simulink model "DC_Charging_Sequence_Block_testing"  (R2024b)
settings: Solver=FixedStepDiscrete  StartTime=0.0  StopTime=10.0  FixedStep=0.01  RelTol=1e-3
undefined symbols (not defined in the file or in its folder): CCM, raptor_get_safe_string, raptor_xcp_function
libraries: Raptor_lib x37
(part 2 of 2)

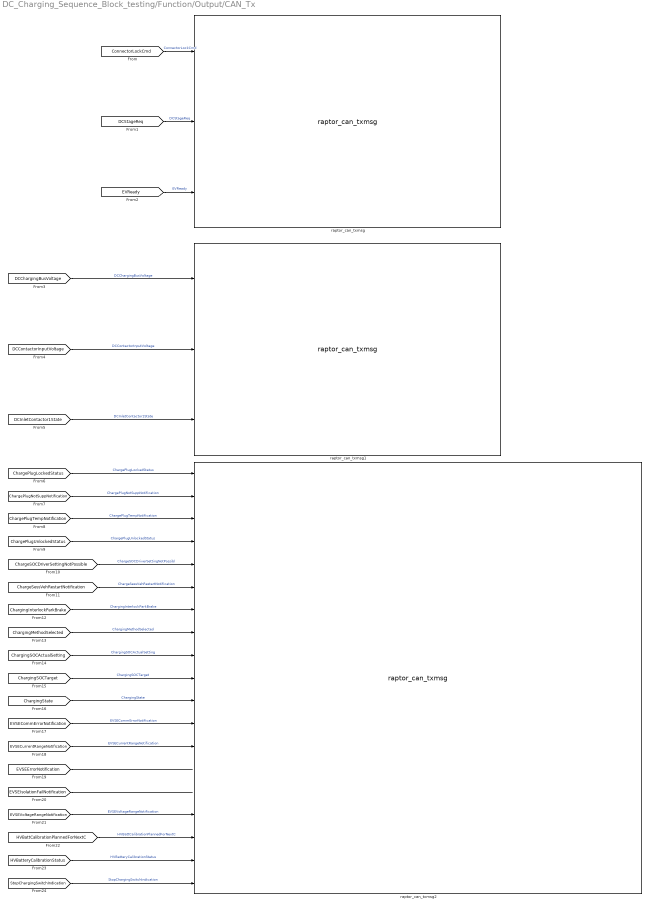
== system DC_Charging_Sequence_Block_testing/Function/Output/CAN_Tx ==
  raptor_can_txmsg : Raptor_lib/CAN/raptor_can_txmsg  canDefinition=struct('dbcFile', 'HCAN_IM40_USETHISONE.dbc','message', 'EVSE1C1_5B','comment', 'EVSE 1 Control 1','signals', {{'ConnectorLockCmd','DCStageReq','EVReady'}},'enabled', [ 1 1 1;],'scaled', [ 1 1 1;],'canBus', '''CAN1''','messageID', [ 408117083;],'idMask', [ 536870911;],'payloadMask', [],'payloadValue', [],'useDbcPeriod', [ 0;],'period', [ 0;],'queueSize', [ 1;],'label', [ 1;],'ver', [ 2;],'showID', [ 0;],'showRaw', [ 0;],'showRawMsg', [ 0;],'useStartVals', [ 0;],'extendedId', [ 1;],'useSimFunc', [ 0;],'sim_func_name', '''''','fill', [ 0;],'editID', [ 0;],'signalOrder', [ 1;],'signalAscDes', [ 1;],'msgLength', [ 8;])  canBus='CAN1'  queueSize=1  payloadMask=[]  payloadValue=[]  period=0  showID=0  label=1  idMask=hex2dec('1FFFFFFF')  fill=0  id=408117083  showRaw=0  signalOrder=1  signalInfo={{struct('Name', 'EVReady','StartBit', [ 8;],'SignalSize', [ 2;],'ByteOrder', 'LittleEndian','ValueType', 'UNSIGNED','Class', 'uint8','Signed', [ 0;],'Factor', [ 1;],'Offset', [ 0;],'Min', [ 0;],'Max', [ 3;],'Units', '','StartVal', [ 0;],'Comment', 'Informs the EVSE that the EV is ready to charge.','Multiplexed', [ 0;],'Multiplexor', [ 0;],'MultiplexMode_Min', [],'MultiplexMode_Max', []),struct('Name', 'DCStageReq','StartBit', [ 4;],'SignalSize', [ 4;],'ByteOrder', 'LittleEndian','ValueType', 'UNSIGNED','Class', 'uint8','Signed', [ 0;],'Factor', [ 1;],'Offset', [ 0;],'Min', [ 0;],'Max', [ 15;],'Units', '','StartVal', [ 0;],'Comment', 'DC EVSE Charging stage request that may be used to cycle the connection to the EVSE through various phases of the charging cycle.','Multiplexed', [ 0;],'Multiplexor', [ 0;],'MultiplexMode_Min', [],'MultiplexMode_Max', []),struct('Name', 'ConnectorLockCmd','StartBit', [ 0;],'SignalSize', [ 4;],'ByteOrder', 'LittleEndian','ValueType', 'UNSIGNED','Class', 'uint8','Signed', [ 0;],'Factor', [ 1;],'Offset', [ 0;],'Min', [ 0;],'Max', [ 15;],'Units', '','StartVal', [ 0;],'Comment', 'Request to engage or disengage the locking mechanism fitted to this EVSE connector to the vehicle.','Multiplexed', [ 0;],'Multiplexor', [ 0;],'MultiplexMode_Min', [],'MultiplexMode_Max', [])}}  useSimFunc=0  sim_func_name=''  useStartVals=0
      settings: SourceProductName=Raptor
  raptor_can_txmsg1 : Raptor_lib/CAN/raptor_can_txmsg  canDefinition=struct('dbcFile', 'HCAN_IM40_USETHISONE.dbc','message', 'EVSE1CS1_5B','comment', 'EVSE 1 Contactor Status 1','signals', {{'DCChargingBusVoltage','DCContactorInputVoltage','DCInletContactor1State'}},'enabled', [ 1 1 1;],'scaled', [ 1 1 1;],'canBus', '''CAN1''','messageID', [ 419084891;],'idMask', [ 536870911;],'payloadMask', [],'payloadValue', [],'useDbcPeriod', [ 0;],'period', [ 0;],'queueSize', [ 1;],'label', [ 1;],'ver', [ 2;],'showID', [ 0;],'showRaw', [ 0;],'showRawMsg', [ 0;],'useStartVals', [ 0;],'extendedId', [ 1;],'useSimFunc', [ 0;],'sim_func_name', '''''','fill', [ 0;],'editID', [ 0;],'signalOrder', [ 1;],'signalAscDes', [ 1;],'msgLength', [ 8;])  canBus='CAN1'  queueSize=1  payloadMask=[]  payloadValue=[]  period=0  showID=0  label=1  idMask=hex2dec('1FFFFFFF')  fill=0  id=419084891  showRaw=0  signalOrder=1  signalInfo={{struct('Name', 'DCInletContactor1State','StartBit', [ 32;],'SignalSize', [ 2;],'ByteOrder', 'LittleEndian','ValueType', 'UNSIGNED','Class', 'uint8','Signed', [ 0;],'Factor', [ 1;],'Offset', [ 0;],'Min', [ 0;],'Max', [ 3;],'Units', '','StartVal', [ 0;],'Comment', 'Indicates the state of DC Inlet Contactor 1.','Multiplexed', [ 0;],'Multiplexor', [ 0;],'MultiplexMode_Min', [],'MultiplexMode_Max', []),struct('Name', 'DCChargingBusVoltage','StartBit', [ 16;],'SignalSize', [ 16;],'ByteOrder', 'LittleEndian','ValueType', 'UNSIGNED','Class', 'uint16','Signed', [ 0;],'Factor', [ 0.05;],'Offset', [ 0;],'Min', [ 0;],'Max', [ 3212.75;],'Units', 'V','StartVal', [ 0;],'Comment', 'Voltage measured on the HVES side of the DC Charging Inlet Contactors.','Multiplexed', [ 0;],'Multiplexor', [ 0;],'MultiplexMode_Min', [],'MultiplexMode_Max', []),struct('Name', 'DCContactorInputVoltage','StartBit', [ 0;],'SignalSize', [ 16;],'ByteOrder', 'LittleEndian','ValueType', 'UNSIGNED','Class', 'uint16','Signed', [ 0;],'Factor', [ 0.05;],'Offset', [ 0;],'Min', [ 0;],'Max', [ 3212.75;],'Units', 'V','StartVal', [ 0;],'Comment', 'Voltage measured on the inlet side of the DC Charging Inlet Contactors.','Multiplexed', [ 0;],'Multiplexor', [ 0;],'MultiplexMode_Min', [],'MultiplexMode_Max', [])}}  useSimFunc=0  sim_func_name=''  useStartVals=0
      settings: SourceProductName=Raptor
  raptor_can_txmsg2 : Raptor_lib/CAN/raptor_can_txmsg  canDefinition=struct('dbcFile', 'HCAN_IM40_USETHISONE.dbc','message', 'HVS_02_5B','comment', 'HVS_02_5B','signals', {{'ChargePlugLockedStatus','ChargePlugNotSuppNotification','ChargePlugTempNotification','ChargePlugUnlockedStatus','ChargeSOCDriverSettingNotPossibl','ChargeSessVehRestartNotification','ChargingInterlockParkBrake','ChargingMethodSelected','ChargingSOCActualSetting','ChargingSOCTarget','ChargingState','EVSECommErrorNotification','EVSECurrentRangeNotification','EVSEErrorNotification','EVSEIsolationFailNotification','EVSEVoltageRangeNotification','HVBattCalibrationPlannedForNextC','HVBatteryCalibrationStatus','StopChargingSwitchIndication'}},'enabled', [ 1 1 1 1 1 1 1 1 1 1 1 1 1 1 1 1 1 1 1;],'scaled', [ 1 1 1 1 1 1 1 1 1 1 1 1 1 1 1 1 1 1 1;],'canBus', '''CAN1''','messageID', [ 419405915;],'idMask', [ 536870911;],'payloadMask', [],'payloadValue', [],'useDbcPeriod', [ 0;],'period', [ 0;],'queueSize', [ 1;],'label', [ 1;],'ver', [ 2;],'showID', [ 0;],'showRaw', [ 0;],'showRawMsg', [ 0;],'useStartVals', [ 0;],'extendedId', [ 1;],'useSimFunc', [ 0;],'sim_func_name', '''''','fill', [ 0;],'editID', [ 0;],'signalOrder', [ 1;],'signalAscDes', [ 1;],'msgLength', [ 8;])  canBus='CAN1'  queueSize=1  payloadMask=[]  payloadValue=[]  period=0  showID=0  label=1  idMask=hex2dec('1FFFFFFF')  fill=0  id=419405915  showRaw=0  signalOrder=1  signalInfo={{struct('Name', 'StopChargingSwitchIndication','StartBit', [ 8;],'SignalSize', [ 2;],'ByteOrder', 'LittleEndian','ValueType', 'UNSIGNED','Class', 'uint8','Signed', [ 0;],'Factor', [ 1;],'Offset', [ 0;],'Min', [ 0;],'Max', [ 0;],'Units', '','StartVal', [ 0;],'Comment', 'StopChargingSwitchIndication','Multiplexed', [ 0;],'Multiplexor', [ 0;],'MultiplexMode_Min', [],'MultiplexMode_Max', []),struct('Name', 'ChargingState','StartBit', [ 0;],'SignalSize', [ 4;],'ByteOrder', 'LittleEndian','ValueType', 'UNSIGNED','Class', 'uint8','Signed', [ 0;],'Factor', [ 1;],'Offset', [ 0;],'Min', [ 0;],'Max', [ 15;],'Units', 'state','StartVal', [ 0;],'Comment', 'ChargingState','Multiplexed', [ 0;],'Multiplexor', [ 0;],'MultiplexMode_Min', [],'MultiplexMode_Max', []),struct('Name', 'ChargePlugLockedStatus','StartBit', [ 4;],'SignalSize', [ 2;],'ByteOrder', 'LittleEndian','ValueType', 'UNSIGNED','Class', 'uint8','Signed', [ 0;],'Factor', [ 1;],'Offset', [ 0;],'Min', [ 0;],'Max', [ 3;],'Units', 'state','StartVal', [ 0;],'Comment', 'ChargePlugLockedStatus','Multiplexed', [ 0;],'Multiplexor', [ 0;],'MultiplexMode_Min', [],'MultiplexMode_Max', []),struct('Name', 'ChargePlugUnlockedStatus','StartBit', [ 6;],'SignalSize', [ 2;],'ByteOrder', 'LittleEndian','ValueType', 'UNSIGNED','Class', 'uint8','Signed', [ 0;],'Factor', [ 1;],'Offset', [ 0;],'Min', [ 0;],'Max', [ 3;],'Units', 'state','StartVal', [ 0;],'Comment', 'ChargePlugUnlockedStatus','Multiplexed', [ 0;],'Multiplexor', [ 0;],'MultiplexMode_Min', [],'MultiplexMode_Max', []),struct('Name', 'ChargePlugNotSuppNotification','StartBit', [ 24;],'SignalSize', [ 2;],'ByteOrder', 'LittleEndian','ValueType', 'UNSIGNED','Class', 'uint8','Signed', [ 0;],'Factor', [ 1;],'Offset', [ 0;],'Min', [ 0;],'Max', [ 3;],'Units', 'state','StartVal', [ 0;],'Comment', 'ChargePlugNotSupportedNotification','Multiplexed', [ 0;],'Multiplexor', [ 0;],'MultiplexMode_Min', [],'MultiplexMode_Max', []),struct('Name', 'ChargePlugTempNotification','StartBit', [ 26;],'SignalSize', [ 2;],'ByteOrder', 'LittleEndian','ValueType', 'UNSIGNED','Class', 'uint8','Signed', [ 0;],'Factor', [ 1;],'Offset', [ 0;],'Min', [ 0;],'Max', [ 3;],'Units', 'state','StartVal', [ 0;],'Comment', 'ChargePlugTemperatureNotification','Multiplexed', [ 0;],'Multiplexor', [ 0;],'MultiplexMode_Min', [],'MultiplexMode_Max', []),struct('Name', 'ChargingInterlockParkBrake','StartBit', [ 28;],'SignalSize', [ 2;],'ByteOrder', 'LittleEndian','ValueType', 'UNSIGNED','Class', 'uint8','Signed', [ 0;],'Factor', [ 1;],'Offset', [ 0;],'Min', [ 0;],'Max', [ 3;],'Units', 'state','StartVal', [ 0;],'Comment', 'ChargingInterlockParkBrake','Multiplexed', [ 0;],'Multiplexor', [ 0;],'MultiplexMode_Min', [],'MultiplexMode_Max', []),struct('Name', 'EVSEErrorNotification','StartBit', [ 30;],'SignalSize', [ 2;],'ByteOrder', 'LittleEndian','ValueType', 'UNSIGNED','Class', 'uint8','Signed', [ 0;],'Factor', [ 1;],'Offset', [ 0;],'Min', [ 0;],'Max', [ 3;],'Units', 'state','StartVal', [ 0;],'Comment', 'EVSEErrorNotification','Multiplexed', [ 0;],'Multiplexor', [ 0;],'MultiplexMode_Min', [],'MultiplexMode_Max', []),struct('Name', 'EVSECommErrorNotification','StartBit', [ 32;],'SignalSize', [ 2;],'ByteOrder', 'LittleEndian','ValueType', 'UNSIGNED','Class', 'uint8','Signed', [ 0;],'Factor', [ 1;],'Offset', [ 0;],'Min', [ 0;],'Max', [ 3;],'Units', 'state','StartVal', [ 0;],'Comment', 'EVSECommunicationErrorNotification','Multiplexed', [ 0;],'Multiplexor', [ 0;],'MultiplexMode_Min', [],'MultiplexMode_Max', []),struct('Name', 'EVSEVoltageRangeNotification','StartBit', [ 34;],'SignalSize', [ 2;],'ByteOrder', 'LittleEndian','ValueType', 'UNSIGNED','Class', 'uint8','Signed', [ 0;],'Factor', [ 1;],'Offset', [ 0;],'Min', [ 0;],'Max', [ 3;],'Units', 'state','StartVal', [ 0;],'Comment', 'EVSEVoltageRangeNotification','Multiplexed', [ 0;],'Multiplexor', [ 0;],'MultiplexMode_Min', [],'MultiplexMode_Max', []),struct('Name', 'EVSECurrentRangeNotification','StartBit', [ 36;],'SignalSize', [ 2;],'ByteOrder', 'LittleEndian','ValueType', 'UNSIGNED','Class', 'uint8','Signed', [ 0;],'Factor', [ 1;],'Offset', [ 0;],'Min', [ 0;],'Max', [ 3;],'Units', 'state','StartVal', [ 0;],'Comment', 'EVSECurrentRangeNotification','Multiplexed', [ 0;],'Multiplexor', [ 0;],'MultiplexMode_Min', [],'MultiplexMode_Max', []),struct('Name', 'EVSEIsolationFailNotification','StartBit', [ 38;],'SignalSize', [ 2;],'ByteOrder', 'LittleEndian','ValueType', 'UNSIGNED','Class', 'uint8','Signed', [ 0;],'Factor', [ 1;],'Offset', [ 0;],'Min', [ 0;],'Max', [ 3;],'Units', 'state','StartVal', [ 0;],'Comment', 'EVSEIsolationFailureNotification','Multiplexed', [ 0;],'Multiplexor', [ 0;],'MultiplexMode_Min', [],'MultiplexMode_Max', []),struct('Name', 'ChargeSessVehRestartNotification','StartBit', [ 40;],'SignalSize', [ 2;],'ByteOrder', 'LittleEndian','ValueType', 'UNSIGNED','Class', 'uint8','Signed', [ 0;],'Factor', [ 1;],'Offset', [ 0;],'Min', [ 0;],'Max', [ 3;],'Units', 'state','StartVal', [ 0;],'Comment', 'ChargingSessionVehicleRestartNotification','Multiplexed', [ 0;],'Multiplexor', [ 0;],'MultiplexMode_Min', [],'MultiplexMode_Max', []),struct('Name', 'HVBatteryCalibrationStatus','StartBit', [ 42;],'SignalSize', [ 2;],'ByteOrder', 'LittleEndian','ValueType', 'UNSIGNED','Class', 'uint8','Signed', [ 0;],'Factor', [ 1;],'Offset', [ 0;],'Min', [ 0;],'Max', [ 3;],'Units', 'state','StartVal', [ 0;],'Comment', 'HighVoltageBatteryCalibrationStatus','Multiplexed', [ 0;],'Multiplexor', [ 0;],'MultiplexMode_Min', [],'MultiplexMode_Max', []),struct('Name', 'HVBattCalibrationPlannedForNextC','StartBit', [ 44;],'SignalSize', [ 2;],'ByteOrder', 'LittleEndian','ValueType', 'UNSIGNED','Class', 'uint8','Signed', [ 0;],'Factor', [ 1;],'Offset', [ 0;],'Min', [ 0;],'Max', [ 3;],'Units', 'state','StartVal', [ 0;],'Comment', 'HighVoltageBatteryCalibrationPlannedforNextCharging','Multiplexed', [ 0;],'Multiplexor', [ 0;],'MultiplexMode_Min', [],'MultiplexMode_Max', []),struct('Name', 'ChargingSOCActualSetting','StartBit', [ 48;],'SignalSize', [ 4;],'ByteOrder', 'LittleEndian','ValueType', 'UNSIGNED','Class', 'uint8','Signed', [ 0;],'Factor', [ 1;],'Offset', [ 0;],'Min', [ 0;],'Max', [ 15;],'Units', 'state','StartVal', [ 0;],'Comment', 'ChargingSOCActualSetting','Multiplexed', [ 0;],'Multiplexor', [ 0;],'MultiplexMode_Min', [],'MultiplexMode_Max', []),struct('Name', 'ChargeSOCDriverSettingNotPossibl','StartBit', [ 52;],'SignalSize', [ 2;],'ByteOrder', 'LittleEndian','ValueType', 'UNSIGNED','Class', 'uint8','Signed', [ 0;],'Factor', [ 1;],'Offset', [ 0;],'Min', [ 0;],'Max', [ 3;],'Units', 'state','StartVal', [ 0;],'Comment', 'ChargingSOCDriverSettingNotPossibleIndication','Multiplexed', [ 0;],'Multiplexor', [ 0;],'MultiplexMode_Min', [],'MultiplexMode_Max', []),struct('Name', 'ChargingMethodSelected','StartBit', [ 54;],'SignalSize', [ 2;],'ByteOrder', 'LittleEndian','ValueType', 'UNSIGNED','Class', 'uint8','Signed', [ 0;],'Factor', [ 1;],'Offset', [ 0;],'Min', [ 0;],'Max', [ 3;],'Units', 'state','StartVal', [ 0;],'Comment', 'ChargingMethodSelected','Multiplexed', [ 0;],'Multiplexor', [ 0;],'MultiplexMode_Min', [],'MultiplexMode_Max', []),struct('Name', 'ChargingSOCTarget','StartBit', [ 56;],'SignalSize', [ 8;],'ByteOrder', 'LittleEndian','ValueType', 'UNSIGNED','Class', 'uint8','Signed', [ 0;],'Factor', [ 0.5;],'Offset', [ 0;],'Min', [ 0;],'Max', [ 125;],'Units', '%','StartVal', [ 0;],'Comment', 'ChargingSOCTarget','Multiplexed', [ 0;],'Multiplexor', [ 0;],'MultiplexMode_Min', [],'MultiplexMode_Max', [])}}  useSimFunc=0  sim_func_name=''  useStartVals=0
      settings: SourceProductName=Raptor
  wires:
  [ConnectorLockCmd] -> raptor_can_txmsg/1  "ConnectorLockCmd"
  [DCStageReq] -> raptor_can_txmsg/2  "DCStageReq"
  [EVReady] -> raptor_can_txmsg/3  "EVReady"
  [DCChargingBusVoltage] -> raptor_can_txmsg1/1  "DCChargingBusVoltage"
  [DCContactorInputVoltage] -> raptor_can_txmsg1/2  "DCContactorInputVoltage"
  [DCInletContactor1State] -> raptor_can_txmsg1/3  "DCInletContactor1State"
  [ChargePlugLockedStatus] -> raptor_can_txmsg2/1  "ChargePlugLockedStatus"
  [ChargePlugNotSuppNotification] -> raptor_can_txmsg2/2  "ChargePlugNotSuppNotification"
  [ChargePlugTempNotification] -> raptor_can_txmsg2/3  "ChargePlugTempNotification"
  [EVSEErrorNotification] -> ?
  [EVSEIsolationFailNotification] -> ?
  [EVSEVoltageRangeNotification] -> raptor_can_txmsg2/16  "EVSEVoltageRangeNotification"
  [HVBattCalibrationPlannedForNextC] -> raptor_can_txmsg2/17  "HVBattCalibrationPlannedForNextC"
  [HVBatteryCalibrationStatus] -> raptor_can_txmsg2/18  "HVBatteryCalibrationStatus"
  [StopChargingSwitchIndication] -> raptor_can_txmsg2/19  "StopChargingSwitchIndication"
  [ChargePlugUnlockedStatus] -> raptor_can_txmsg2/4  "ChargePlugUnlockedStatus"
  [ChargeSOCDriverSettingNotPossible] -> raptor_can_txmsg2/5  "ChargeSOCDriverSettingNotPossibl"
  [ChargeSessVehRestartNotification] -> raptor_can_txmsg2/6  "ChargeSessVehRestartNotification"
  [ChargingInterlockParkBrake] -> raptor_can_txmsg2/7  "ChargingInterlockParkBrake"
  [ChargingMethodSelected] -> raptor_can_txmsg2/8  "ChargingMethodSelected"
  [ChargingSOCActualSetting] -> raptor_can_txmsg2/9  "ChargingSOCActualSetting"
  [ChargingSOCTarget] -> raptor_can_txmsg2/10  "ChargingSOCTarget"
  [ChargingState] -> raptor_can_txmsg2/11  "ChargingState"
  [EVSECommErrorNotification] -> raptor_can_txmsg2/12  "EVSECommErrorNotification"
  [EVSECurrentRangeNotification] -> raptor_can_txmsg2/13  "EVSECurrentRangeNotification"

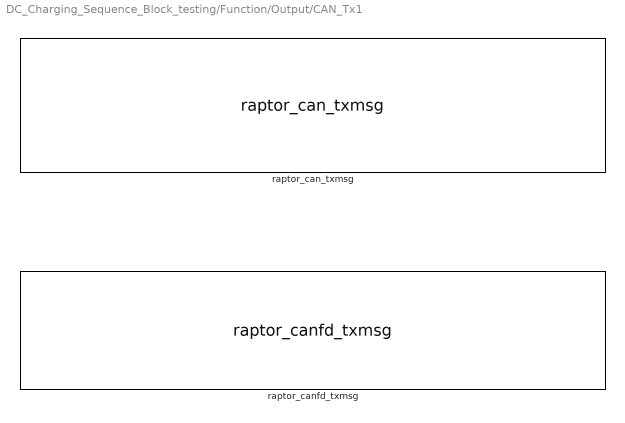
== system DC_Charging_Sequence_Block_testing/Function/Output/CAN_Tx1 ==
  raptor_can_txmsg : Raptor_lib/CAN/raptor_can_txmsg  canDefinition=struct('dbcFile', '.\CAN\can_example.dbc','message', 'ExampleMsgTxExtended','comment', '','signals', {{'Enable','EngineSpeed','EngineTemperature'}},'enabled', [ 1 1 1;],'canBus', '''CAN1''','messageID', [ 777;],'idMask', [ 536870911;],'payloadMask', [],'payloadValue', [],'period', [ 0;],'mailbox', '','queueSize', [ 1;],'label', [ 0;],'ver', [ 2;],'showID', [ 0;],'showRaw', [ 0;],'fill', [ 0;],'editID', [ 0;],'signalOrder', [ 1;])  canBus='CAN1'  queueSize=1  payloadMask=[]  payloadValue=[]  period=0  showID=0  label=0  idMask=hex2dec('1FFFFFFF')  fill=0  id=777  showRaw=0  signalOrder=1  signalInfo={{struct('Name', 'Enable','StartBit', [ 0;],'SignalSize', [ 1;],'ByteOrder', 'BigEndian','ValueType', 'UNSIGNED','Class', 'uint8','Signed', [ 0;],'Factor', [ 1;],'Offset', [ 0;],'Min', [ 0;],'Max', [ 1;],'Units', '','StartVal', [ 0;],'Comment', '','Multiplexed', [ 0;],'Multiplexor', [ 0;],'MultiplexMode_Min', [],'MultiplexMode_Max', []),struct('Name', 'EngineSpeed','StartBit', [ 16;],'SignalSize', [ 16;],'ByteOrder', 'BigEndian','ValueType', 'UNSIGNED','Class', 'uint16','Signed', [ 0;],'Factor', [ 0.1;],'Offset', [ 0;],'Min', [ 0;],'Max', [ 6500;],'Units', 'rpm','StartVal', [ 0;],'Comment', '','Multiplexed', [ 0;],'Multiplexor', [ 0;],'MultiplexMode_Min', [],'MultiplexMode_Max', []),struct('Name', 'EngineTemperature','StartBit', [ 32;],'SignalSize', [ 16;],'ByteOrder', 'BigEndian','ValueType', 'UNSIGNED','Class', 'uint16','Signed', [ 0;],'Factor', [ 0.01;],'Offset', [ -40;],'Min', [ -40;],'Max', [ 500;],'Units', 'degC','StartVal', [ 0;],'Comment', '','Multiplexed', [ 0;],'Multiplexor', [ 0;],'MultiplexMode_Min', [],'MultiplexMode_Max', [])}}  useSimFunc=0  sim_func_name=''  useStartVals=0
      settings: SourceProductName=Raptor
  raptor_canfd_txmsg : Raptor_lib/CAN/raptor_canfd_txmsg  canDefinition=struct('dbcFile', '.\CAN\can_example.dbc','message', 'ExampleMsgTxExtended','comment', '','signals', {{'Enable','EngineSpeed','EngineTemperature'}},'enabled', [ 1 1 1;],'canBus', '''CAN1''','messageID', [ 777;],'idMask', [ 536870911;],'payloadMask', [],'payloadValue', [],'period', [ 0;],'mailbox', '','queueSize', [ 1;],'label', [ 0;],'ver', [ 2;],'showID', [ 0;],'showRaw', [ 0;],'fill', [ 0;],'editID', [ 0;],'signalOrder', [ 1;])  canBus='CAN1'  queueSize=1  payloadMask=[]  payloadValue=[]  period=0  showID=0  label=0  idMask=hex2dec('1FFFFFFF')  fill=0  id=777  showRaw=0  signalOrder=1  signalInfo={{struct('Name', 'Enable','StartBit', [ 0;],'SignalSize', [ 1;],'ByteOrder', 'BigEndian','ValueType', 'UNSIGNED','Class', 'uint8','Signed', [ 0;],'Factor', [ 1;],'Offset', [ 0;],'Min', [ 0;],'Max', [ 1;],'Units', '','StartVal', [ 0;],'Comment', '','Multiplexed', [ 0;],'Multiplexor', [ 0;],'MultiplexMode_Min', [],'MultiplexMode_Max', []),struct('Name', 'EngineSpeed','StartBit', [ 16;],'SignalSize', [ 16;],'ByteOrder', 'BigEndian','ValueType', 'UNSIGNED','Class', 'uint16','Signed', [ 0;],'Factor', [ 0.1;],'Offset', [ 0;],'Min', [ 0;],'Max', [ 6500;],'Units', 'rpm','StartVal', [ 0;],'Comment', '','Multiplexed', [ 0;],'Multiplexor', [ 0;],'MultiplexMode_Min', [],'MultiplexMode_Max', []),struct('Name', 'EngineTemperature','StartBit', [ 32;],'SignalSize', [ 16;],'ByteOrder', 'BigEndian','ValueType', 'UNSIGNED','Class', 'uint16','Signed', [ 0;],'Factor', [ 0.01;],'Offset', [ -40;],'Min', [ -40;],'Max', [ 500;],'Units', 'degC','StartVal', [ 0;],'Comment', '','Multiplexed', [ 0;],'Multiplexor', [ 0;],'MultiplexMode_Min', [],'MultiplexMode_Max', [])}}  useSimFunc=0  sim_func_name=''  useStartVals=0  brsEnable=0  fdEnable=false
      settings: SourceProductName=Raptor

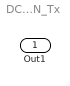
== system DC_Charging_Sequence_Block_testing/Function/Output/LIN_Tx ==
  Out1 : Outport
  wires:
  ? -> Out1/1
